simulink model "questao9_final"  (R2023a)
settings: Solver=VariableStepAuto  StartTime=0.0  StopTime=30  RelTol=1e-3
libraries: slpidlib x2
settings Model: Creator=13199959938  LastModifiedBy=mluser
settings SolverCC: AlgebraicLoopSolver=TrustRegion
settings DataIOCC: ReturnWorkspaceOutputs=off
settings OptimizationCC: ReuseModelBlockBuffer=off
settings DebuggingCC: UnconnectedInputMsg=warning  UnconnectedOutputMsg=warning  UnconnectedLineMsg=warning  ArithmeticOperatorsInVariantConditions=warning
settings ModelReferenceCC: EnableRefExpFcnMdlSchedulingChecks=on
settings SFSimCC: SimUseLocalCustomCode=off  CustomCodeUndefinedFunction=UseInterfaceOnly
settings RTWCC: RTWUseLocalCustomCode=off
settings CodeAppCC: StateflowObjectComments=on

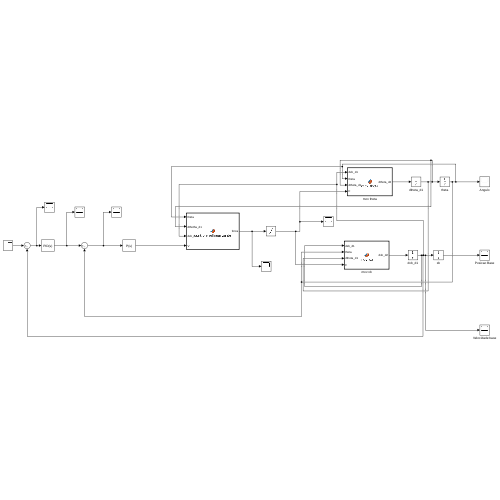
[thumbnail: Simulink's stored preview of the top-level diagram]
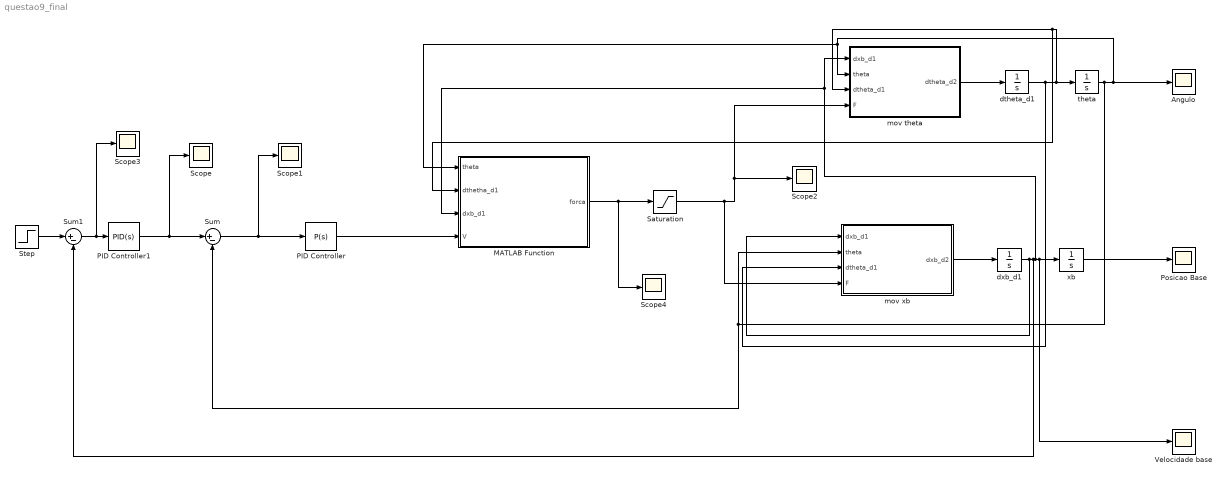
== system questao9_final ==
  Angulo : Scope
  MATLAB Function : MATLAB Function  TreatAsAtomicUnit=on
  PID Controller : slpidlib/PID Controller  Controller=P  Form=Parallel  TimeDomain=Continuous-time  UseExternalTs=off  SampleTime=-1  IntegratorMethod=Forward Euler  FilterMethod=Forward Euler  ControllerParametersSource=internal  P=1250  I=450  UseKiTs=off  D=0  N=100  UseFilter=on  TunerSelectOption=Transfer Function Based (PID Tuner App)  InitialConditionSource=internal  InitialConditionForIntegrator=0  InitialConditionForFilter=0  DifferentiatorICPrevScaledInput=0  ExternalReset=none  TrackingMode=off  Kt=1  LimitOutput=off  SatLimitsSource=internal  UpperSaturationLimit=inf  LowerSaturationLimit=-inf  LinearizeAsGain=on  AntiWindupMode=none  Kb=1  LimitIntegrator=off  UpperIntegratorSaturationLimit=inf  LowerIntegratorSaturationLimit=-inf  POutMin=[]  POutMax=[]  IOutMin=[]  IOutMax=[]  DOutMin=[]  DOutMax=[]  NOutMin=[]  NOutMax=[]  SumOutMin=[]  SumOutMax=[]  SaturationOutMin=[]  SaturationOutMax=[]  PParamMin=[]  PParamMax=[]  IParamMin=[]  IParamMax=[]  DParamMin=[]  DParamMax=[]  NParamMin=[]  NParamMax=[]  KbParamMin=[]  KbParamMax=[]  KtParamMin=[]  KtParamMax=[]  KbOutMin=[]  KbOutMax=[]  KtOutMin=[]  KtOutMax=[]  IntegratorOutMin=[]  IntegratorOutMax=[]  FilterOutMin=[]  FilterOutMax=[]  SumI1OutMin=[]  SumI1OutMax=[]  SumI2OutMin=[]  SumI2OutMax=[]  SumI3OutMin=[]  SumI3OutMax=[]  SumI4OutMin=[]  SumI4OutMax=[]  SumDOutMin=[]  SumDOutMax=[]  DifferentiatorOutMin=[]  DifferentiatorOutMax=[]  FilterDiffOutCoefMin=[]  FilterDiffOutCoefMax=[]  ReciprocalOutMin=[]  ReciprocalOutMax=[]  SumDenOutMin=[]  SumDenOutMax=[]  SumNumOutMin=[]  SumNumOutMax=[]  DivideOutMin=[]  DivideOutMax=[]  UdiffTsProdOutMin=[]  UdiffTsProdOutMax=[]  NTsProdOutMin=[]  NTsProdOutMax=[]  UintegralTsProdOutMin=[]  UintegralTsProdOutMax=[]  UngainTsProdOutMin=[]  UngainTsProdOutMax=[]  ClampingZeroOutDataTypeStr=Inherit: Inherit via back propagation  ClampingZeroOutMin=[]  ClampingZeroOutMax=[]  FilterDenConstantOutDataTypeStr=Inherit: Inherit via back propagation  FilterDenConstantOutMin=[]  FilterDenConstantOutMax=[]  PCopyOutDataTypeStr=Inherit: Inherit via back propagation  PCopyOutMin=[]  PCopyOutMax=[]  NCopyOutDataTypeStr=Inherit: Inherit via back propagation  NCopyOutMin=[]  NCopyOutMax=[]  IntegratorContinuousStateAttributes=''  IntegratorStateMustResolveToSignalObject=off  IntegratorRTWStateStorageClass=Auto  FilterContinuousStateAttributes=''  FilterStateMustResolveToSignalObject=off  FilterRTWStateStorageClass=Auto  ParallelPVariant=InternalParameters  IdealPVariant=Disabled  IVariant=Disabled  DVariant=Disabled  IntegratorVariant=Disabled  SatVariant=Disabled  AWVariant=Disabled  PCopyVariant=Disabled  TRVariant=Disabled  FdbkBlocksVariant=Forward  IdealPFdbkVariant=Disabled  SatFdbkVariant=Disabled  DerivativeFilterVariant=Disabled  NVariant=Disabled  NCopyVariant=Disabled_SignalSpec  FilterICVariant=Disabled  IntegratorICVariant=Disabled  ExternalResetVariant=Disabled  TRSumVariant=Passthrough  SumFdbkVariant=Disabled  SumVariant=Passthrough_P  TsampFilterVariant=InternalTs  TsampNgainVariant=Passthrough  TsampIntegralVariant=Disabled_SignalSpec  ExternalSaturationOutDataTypeStr=Inherit: Same as second input
  PID Controller1 : slpidlib/PID Controller  Controller=PID  Form=Parallel  TimeDomain=Continuous-time  UseExternalTs=off  SampleTime=-1  IntegratorMethod=Forward Euler  FilterMethod=Forward Euler  ControllerParametersSource=internal  P=-0.056  I=0  UseKiTs=off  D=0.0188  N=2.21  UseFilter=on  TunerSelectOption=Transfer Function Based (PID Tuner App)  InitialConditionSource=internal  InitialConditionForIntegrator=0  InitialConditionForFilter=0  DifferentiatorICPrevScaledInput=0  ExternalReset=none  TrackingMode=off  Kt=1  LimitOutput=off  SatLimitsSource=internal  UpperSaturationLimit=inf  LowerSaturationLimit=-inf  LinearizeAsGain=on  AntiWindupMode=none  Kb=1  LimitIntegrator=off  UpperIntegratorSaturationLimit=inf  LowerIntegratorSaturationLimit=-inf  POutMin=[]  POutMax=[]  IOutMin=[]  IOutMax=[]  DOutMin=[]  DOutMax=[]  NOutMin=[]  NOutMax=[]  SumOutMin=[]  SumOutMax=[]  SaturationOutMin=[]  SaturationOutMax=[]  PParamMin=[]  PParamMax=[]  IParamMin=[]  IParamMax=[]  DParamMin=[]  DParamMax=[]  NParamMin=[]  NParamMax=[]  KbParamMin=[]  KbParamMax=[]  KtParamMin=[]  KtParamMax=[]  KbOutMin=[]  KbOutMax=[]  KtOutMin=[]  KtOutMax=[]  IntegratorOutMin=[]  IntegratorOutMax=[]  FilterOutMin=[]  FilterOutMax=[]  SumI1OutMin=[]  SumI1OutMax=[]  SumI2OutMin=[]  SumI2OutMax=[]  SumI3OutMin=[]  SumI3OutMax=[]  SumI4OutMin=[]  SumI4OutMax=[]  SumDOutMin=[]  SumDOutMax=[]  DifferentiatorOutMin=[]  DifferentiatorOutMax=[]  FilterDiffOutCoefMin=[]  FilterDiffOutCoefMax=[]  ReciprocalOutMin=[]  ReciprocalOutMax=[]  SumDenOutMin=[]  SumDenOutMax=[]  SumNumOutMin=[]  SumNumOutMax=[]  DivideOutMin=[]  DivideOutMax=[]  UdiffTsProdOutMin=[]  UdiffTsProdOutMax=[]  NTsProdOutMin=[]  NTsProdOutMax=[]  UintegralTsProdOutMin=[]  UintegralTsProdOutMax=[]  UngainTsProdOutMin=[]  UngainTsProdOutMax=[]  ClampingZeroOutDataTypeStr=Inherit: Inherit via back propagation  ClampingZeroOutMin=[]  ClampingZeroOutMax=[]  FilterDenConstantOutDataTypeStr=Inherit: Inherit via back propagation  FilterDenConstantOutMin=[]  FilterDenConstantOutMax=[]  PCopyOutDataTypeStr=Inherit: Inherit via back propagation  PCopyOutMin=[]  PCopyOutMax=[]  NCopyOutDataTypeStr=Inherit: Inherit via back propagation  NCopyOutMin=[]  NCopyOutMax=[]  IntegratorContinuousStateAttributes=''  IntegratorStateMustResolveToSignalObject=off  IntegratorRTWStateStorageClass=Auto  FilterContinuousStateAttributes=''  FilterStateMustResolveToSignalObject=off  FilterRTWStateStorageClass=Auto  ParallelPVariant=InternalParameters  IdealPVariant=Disabled  IVariant=InternalParameters  DVariant=InternalParameters  IntegratorVariant=Continuous  SatVariant=Disabled  AWVariant=Passthrough  PCopyVariant=Disabled  TRVariant=Disabled  FdbkBlocksVariant=Forward  IdealPFdbkVariant=Disabled  SatFdbkVariant=Disabled  DerivativeFilterVariant=ContFilter  NVariant=InternalParameters  NCopyVariant=Disabled  FilterICVariant=InternalICsFilter  IntegratorICVariant=InternalICs  ExternalResetVariant=Disabled  TRSumVariant=Passthrough  SumFdbkVariant=Disabled  SumVariant=Sum_PID  TsampFilterVariant=InternalTs  TsampNgainVariant=Passthrough  TsampIntegralVariant=Disabled_SignalSpec  ExternalSaturationOutDataTypeStr=Inherit: Same as second input
  Posicao Base : Scope
  Saturation : Saturate  UpperLimit=540  LowerLimit=-540
  Scope{,1..4} (5 alike) : Scope
  Step : Step  Time=0  After=2  SampleTime=0
  Sum : Sum  Inputs=|+-
  Sum1 : Sum  Inputs=|+-
  Velocidade base : Scope
  dtheta_d1 : Integrator
  dxb_d1 : Integrator
  mov theta : MATLAB Function  TreatAsAtomicUnit=on
  mov xb : MATLAB Function  TreatAsAtomicUnit=on
  theta : Integrator
  xb : Integrator
  wires:
  mov xb/1(dxb_d2) -> dxb_d1/1
  mov theta/1(dtheta_d2) -> dtheta_d1/1
  dtheta_d1/1 -> mov xb/3(dtheta_d1), MATLAB Function/2(dthetha_d1), mov theta/3(dtheta_d1), theta/1
  theta/1 -> Sum/2, mov xb/2(theta), Angulo/1, mov theta/2(theta), MATLAB Function/1(theta)
  dxb_d1/1 -> mov xb/1(dxb_d1), xb/1, Velocidade base/1, mov theta/1(dxb_d1), MATLAB Function/3(dxb_d1), Sum1/2
  xb/1 -> Posicao Base/1
  MATLAB Function/1(forca) -> Scope4/1, Saturation/1
  Saturation/1 -> mov xb/4(F), mov theta/4(F), Scope2/1
  Sum/1 -> Scope1/1, PID Controller/1
  PID Controller/1 -> MATLAB Function/4(V)
  PID Controller1/1 -> Scope/1, Sum/1
  Sum1/1 -> Scope3/1, PID Controller1/1
  Step/1 -> Sum1/1

== matlab function questao9_final/mov xb ==
  data: dxb_d1 input; dxb_d2 output; theta input; dtheta_d1 input; F input
function dxb_d2 = mov_xb(dxb_d1, theta, dtheta_d1, F)
    g = 9.81; % m/s^2
    l = 1.30; % m
    m = 60; % kg
    M = 54; % kg
    b = 130; % atrito viscoso com o ar
    d = 97.2; % Ns/M
    
    dxb_d2 = (F-d*dxb_d1-m*l*sin(theta)*dtheta_d1^2+m*g*sin(theta)*cos(theta)-(b*dtheta_d1*cos(theta))/l)/((M+m*(sin(theta))^2));

== matlab function questao9_final/mov theta ==
  data: dxb_d1 input; dtheta_d2 output; theta input; dtheta_d1 input; F input
function dtheta_d2 = mov_theta(dxb_d1, theta, dtheta_d1, F)
    g = 9.81; % m/s^2
    l = 1.30; % m
    m = 60; % kg
    M = 54; % kg
    b = 130; % atrito viscoso com o ar
    d = 97.2; % Ns/M
    
    dtheta_d2 = ((M+m)*g*l*sin(theta)+l*cos(theta)*(F-d*dxb_d1-m*l*sin(theta)*dtheta_d1^2)-((M+m)*b*dtheta_d1)/m)/(l^2*(M+m*(sin(theta))^2));

== matlab function questao9_final/MATLAB Function ==
  data: theta input; forca output; dthetha_d1 input; dxb_d1 input; V input
function forca = controle_relinearizante(theta, dthetha_d1, dxb_d1, V)
    g = 9.81; % m/s^2
    l = 1.30; % m
    m = 60; % kg
    M = 54; % kg
    b = 130; % atrito viscoso com o ar
    d = 97.2; % Ns/M

   % forca = (-(M+m)*l*g*sin(theta) +m*l^2*sin(theta)*cos(theta)*dtheta_d1^2 + d*l*cos(theta)*dxb_d1+V) / (l*cos(theta));
   %forca = (((V - ((M+m)*b*dtheta_d1)/m)*l^2*(M+m*(sin(theta))^2))/(M*l^2)- (M+m)*g*l*sin(theta)+m*l^2*sin(theta)*cos(theta)*dtheta_d1^2+d*l*cos(theta)*dxb_d1+((M+m)*b*dtheta_d1)/m )/(l*cos(theta));
   forca =(-b*m*dthetha_d1*sin(theta)* tan(theta) - b *M *dthetha_d1* sin(theta) *tan(theta) + d *l *M* dxb_d1 - g* l *m *M* tan(theta) - g *l *M^2 *tan(theta) + l^2* m* M* dthetha_d1^2 *sin(theta) + m* V *sin(theta)* tan(theta) + M *V* sec(theta))/(l* M); %and l*M!=0 and m^2*sin^2(t)*cos(t) + m*M*cos(t)!=0
